simulink model "Exp5_simulink"  (R2019b)
settings: Solver=VariableStepAuto  StartTime=0.0  StopTime=0.8  RelTol=1e-3
undefined symbols (not defined in the file): Pm, Pm2, Pm3
settings Model: Creator=admin  LastModifiedBy=admin

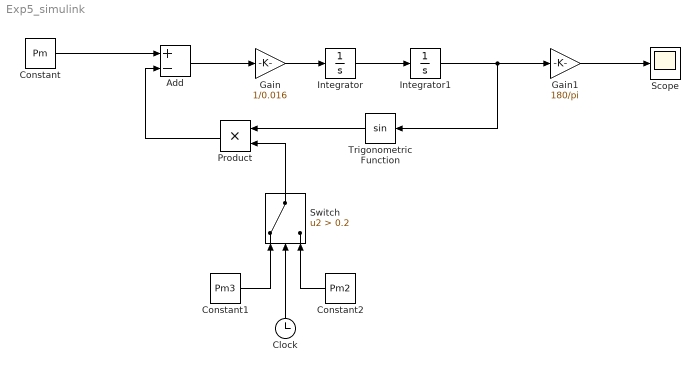
== system Exp5_simulink ==
  Add : Sum  Inputs=+-
  Clock : Clock
  Constant : Constant  Value=Pm
  Constant1 : Constant  Value=Pm3
  Constant2 : Constant  Value=Pm2
  Gain : Gain  Gain=1/0.016
  Gain1 : Gain  Gain=180/pi
  Integrator : Integrator
  Integrator1 : Integrator
  Product : Product
  Scope : Scope
  Switch : Switch  Criteria=u2 > Threshold  Threshold=0.2
  Trigonometric Function : Trigonometry
  wires:
  Constant1/1 -> Switch/1
  Clock/1 -> Switch/2
  Constant2/1 -> Switch/3
  Constant/1 -> Add/1
  Add/1 -> Gain/1
  Gain/1 -> Integrator/1
  Integrator/1 -> Integrator1/1
  Integrator1/1 -> Trigonometric Function/1, Gain1/1
  Switch/1 -> Product/2
  Product/1 -> Add/2
  Trigonometric Function/1 -> Product/1
  Gain1/1 -> Scope/1
